simulink model "solver"  (R2022b)
settings: Solver=ode45  StartTime=0.0  StopTime=15.0  MaxStep=0.05  RelTol=1e-3
values from neighbouring files (symbols this model uses):
  Jb11 = m*(b^2+c^2)/12    (= 8.33333333333e-09)    [startup.m]
  Jb22 = m*(a^2+c^2)/12    (= 7.08333333333e-09)    [startup.m]
  Jb33 = m*(a^2+b^2)/12    (= 2.08333333333e-09)    [startup.m]
  Wx = Wxtilde*sqrt(0.99)    [startup.m]
  Wxtilde = sqrt((2*K)/Jb11)    [startup.m]
  Wy = Wytilde*sqrt(0.99)    [startup.m]
  Wz = Wztilde*sqrt(0.99)    [startup.m]
  Wztilde = 2*pi    (= 6.28318530718)    [startup.m]
libraries: vrlib x3
settings Model: Creator=eleves  LastModifiedBy=eleves

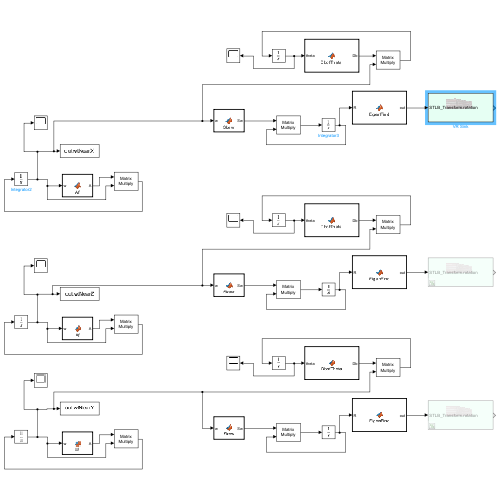
[thumbnail: Simulink's stored preview of the top-level diagram]
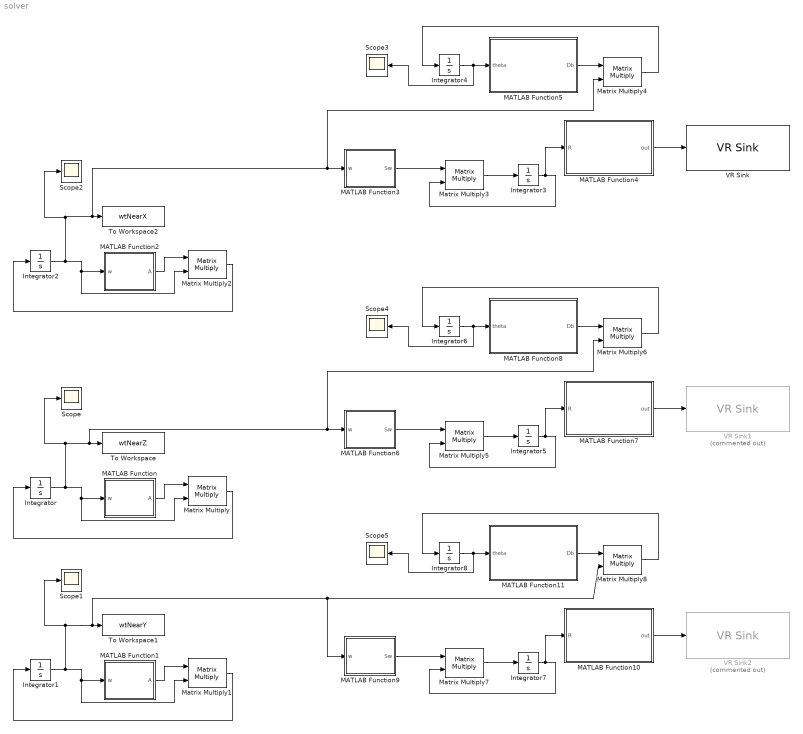
== system solver ==
  Integrator : Integrator  InitialCondition=[Wxtilde/10;0;Wz]
  Integrator1 : Integrator  InitialCondition=[0;Wy;Wztilde/10]
  Integrator2 : Integrator  InitialCondition=[Wx;0;Wztilde/10]
  Integrator3 : Integrator  InitialCondition=[1,0,0; 0,1,0; 0,0,1]
  Integrator4 : Integrator  InitialCondition=[0;0;0]
  Integrator5 : Integrator  InitialCondition=[1,0,0; 0,1,0; 0,0,1]
  Integrator6 : Integrator  InitialCondition=[0;0;0]
  Integrator7 : Integrator  InitialCondition=[1,0,0; 0,1,0; 0,0,1]
  Integrator8 : Integrator  InitialCondition=[0;0;0]
  MATLAB Function : MATLAB Function  TreatAsAtomicUnit=on
  MATLAB Function1 : MATLAB Function  TreatAsAtomicUnit=on
  MATLAB Function10 : MATLAB Function  TreatAsAtomicUnit=on
  MATLAB Function11 : MATLAB Function  TreatAsAtomicUnit=on
  MATLAB Function2 : MATLAB Function  TreatAsAtomicUnit=on
  MATLAB Function3 : MATLAB Function  TreatAsAtomicUnit=on
  MATLAB Function4 : MATLAB Function  TreatAsAtomicUnit=on
  MATLAB Function5 : MATLAB Function  TreatAsAtomicUnit=on
  MATLAB Function6 : MATLAB Function  TreatAsAtomicUnit=on
  MATLAB Function7 : MATLAB Function  TreatAsAtomicUnit=on
  MATLAB Function8 : MATLAB Function  TreatAsAtomicUnit=on
  MATLAB Function9 : MATLAB Function  TreatAsAtomicUnit=on
  Matrix Multiply{,1..8} (9 alike) : Product  Multiplication=Matrix(*)
  Scope{,1..5} (6 alike) : Scope
  To Workspace : ToWorkspace  VariableName=wtNearZ  SaveFormat=Timeseries  SampleTime=-1
  To Workspace1 : ToWorkspace  VariableName=wtNearY  SaveFormat=Timeseries  SampleTime=-1
  To Workspace2 : ToWorkspace  VariableName=wtNearX  SaveFormat=Timeseries  SampleTime=-1
  VR Sink : vrlib/VR Sink  InstantiateOnLoad=on  SampleTime=0.01  ViewEnable=on  RemoteChange=off  RemoteView=off  FieldsWritten=STLB_Transform.rotation.4.1.1.double  WorldFileName=test.x3d  AutoView=off  VideoDimensions=[200 320]  AllowVariableSize=off
  VR Sink1 : vrlib/VR Sink  Commented=on  InstantiateOnLoad=on  SampleTime=0.01  ViewEnable=on  RemoteChange=off  RemoteView=off  FieldsWritten=STLB_Transform.rotation.4.1.1.double  WorldFileName=test.x3d  AutoView=off  VideoDimensions=[200 320]  AllowVariableSize=off
  VR Sink2 : vrlib/VR Sink  Commented=on  InstantiateOnLoad=on  SampleTime=0.01  ViewEnable=on  RemoteChange=off  RemoteView=off  FieldsWritten=STLB_Transform.rotation.4.1.1.double  WorldFileName=test.x3d  AutoView=off  VideoDimensions=[200 320]  AllowVariableSize=off
  wires:
  MATLAB Function/1(A) -> Matrix Multiply/1
  Matrix Multiply/1 -> Integrator/1
  MATLAB Function1/1(A) -> Matrix Multiply1/1
  Matrix Multiply1/1 -> Integrator1/1
  Integrator2/1 -> Matrix Multiply4/2, MATLAB Function3/1(w), To Workspace2/1, Scope2/1, Matrix Multiply2/2, MATLAB Function2/1(w)
  MATLAB Function2/1(A) -> Matrix Multiply2/1
  Matrix Multiply2/1 -> Integrator2/1
  MATLAB Function3/1(Sw) -> Matrix Multiply3/1
  Matrix Multiply3/1 -> Integrator3/1
  Integrator3/1 -> MATLAB Function4/1(R), Matrix Multiply3/2
  MATLAB Function4/1(out) -> VR Sink/1
  Integrator4/1 -> Scope3/1, MATLAB Function5/1(theta)
  MATLAB Function5/1(Db) -> Matrix Multiply4/1
  Matrix Multiply4/1 -> Integrator4/1
  Integrator6/1 -> Scope4/1, MATLAB Function8/1(theta)
  MATLAB Function8/1(Db) -> Matrix Multiply6/1
  Matrix Multiply6/1 -> Integrator6/1
  MATLAB Function7/1(out) -> VR Sink1/1
  Integrator5/1 -> MATLAB Function7/1(R), Matrix Multiply5/2
  Integrator/1 -> Matrix Multiply6/2, MATLAB Function6/1(w), To Workspace/1, Scope/1, Matrix Multiply/2, MATLAB Function/1(w)
  Matrix Multiply5/1 -> Integrator5/1
  MATLAB Function6/1(Sw) -> Matrix Multiply5/1
  Integrator8/1 -> Scope5/1, MATLAB Function11/1(theta)
  MATLAB Function11/1(Db) -> Matrix Multiply8/1
  Matrix Multiply8/1 -> Integrator8/1
  MATLAB Function10/1(out) -> VR Sink2/1
  Integrator7/1 -> MATLAB Function10/1(R), Matrix Multiply7/2
  Integrator1/1 -> MATLAB Function9/1(w), Matrix Multiply8/2, To Workspace1/1, Scope1/1, Matrix Multiply1/2, MATLAB Function1/1(w)
  Matrix Multiply7/1 -> Integrator7/1
  MATLAB Function9/1(Sw) -> Matrix Multiply7/1

== matlab function solver/MATLAB Function1 ==
  data: w input; A output; Jb11 parameter; Jb22 parameter; Jb33 parameter
function A = Af(w, Jb11,Jb22, Jb33)

A = [0, (1/Jb11)*0.5*(Jb22-Jb33)*w(3),(1/Jb11)*0.5*(Jb22-Jb33)*w(2);
    (1/Jb22)*0.5*(Jb33-Jb11)*w(3),0,(1/Jb22)*0.5*(Jb33-Jb11)*w(1);
    (1/Jb33)*0.5*(Jb11-Jb22)*w(2),(1/Jb33)*0.5*(Jb11-Jb22)*w(1),0];

== matlab function solver/MATLAB Function ==
  data: w input; A output; Jb11 parameter; Jb22 parameter; Jb33 parameter
function A = Af(w, Jb11,Jb22, Jb33)

A = [0, (1/Jb11)*0.5*(Jb22-Jb33)*w(3),(1/Jb11)*0.5*(Jb22-Jb33)*w(2);
    (1/Jb22)*0.5*(Jb33-Jb11)*w(3),0,(1/Jb22)*0.5*(Jb33-Jb11)*w(1);
    (1/Jb33)*0.5*(Jb11-Jb22)*w(2),(1/Jb33)*0.5*(Jb11-Jb22)*w(1),0];

== matlab function solver/MATLAB Function2 ==
  data: w input; A output; Jb11 parameter; Jb22 parameter; Jb33 parameter
function A = Af(w, Jb11,Jb22, Jb33)

A = [0, (1/Jb11)*0.5*(Jb22-Jb33)*w(3),(1/Jb11)*0.5*(Jb22-Jb33)*w(2);
    (1/Jb22)*0.5*(Jb33-Jb11)*w(3),0,(1/Jb22)*0.5*(Jb33-Jb11)*w(1);
    (1/Jb33)*0.5*(Jb11-Jb22)*w(2),(1/Jb33)*0.5*(Jb11-Jb22)*w(1),0];

== matlab function solver/MATLAB Function3 ==
  data: w input; Sw output
function Sw = Skew(w)

Sw = [0,-w(3),w(2);
    w(3),0,-w(1);
    -w(2),w(1),0];

== matlab function solver/MATLAB Function4 ==
  data: R input; out output
function out = EigenFind(R)

    epsilon = 0.01; 
    epsilon2 = 0.1;
    
    if (abs(R(0+1,1+1)-R(1+1,0+1))< epsilon) && (abs(R(0+1,2+1)-R(2+1,0+1))< epsilon) && (abs(R(1+1,2+1)-R(2+1,1+1))< epsilon) 
	    % singularity found
	    % first check for identity matrix which must have +1 for all terms
	    %  in leading diagonaland zero in other terms
	    if (abs(R(0+1,1+1)+R(1+1,0+1)) < epsilon2) && (abs(R(0+1,2+1)+R(2+1,0+1)) < epsilon2) && (abs(R(1+1,2+1)+R(2+1,1+1)) < epsilon2) && (abs(R(0+1,0+1)+R(1+1,1+1)+R(2+1,2+1)-3) < epsilon2)
		    % this singularity is identity matrix so angle = 0
		    out= [1,0,0,0]; % zero angle, arbitrary axis
	    end
	    % otherwise this singularity is angle = 180
	    angle = pi;
	    xx = (R(0+1,0+1)+1)/2;
	    yy = (R(1+1,1+1)+1)/2;
	    zz = (R(2+1,2+1)+1)/2;
	    xy = (R(0+1,1+1)+R(1+1,0+1))/4;
	    xz = (R(0+1,2+1)+R(2+1,0+1))/4;
	    yz = (R(1+1,2+1)+R(2+1,1+1))/4;
	    if (xx > yy) && (xx > zz)  % R(0+1,0+1) is the largest diagonal term
		    if (xx< epsilon) 
			    x = 0;
			    y = 0.7071;
			    z = 0.7071;
		    else 
			    x = sqrt(xx);
			    y = xy/x;
			    z = xz/x;
		    end
    
	    elseif (yy > zz)  % R(1+1,1+1) is the largest diagonal term
		    if (yy< epsilon) 
			    x = 0.7071;
			    y = 0;
			    z = 0.7071;
		    else 
			    y = sqrt(yy);
			    x = xy/y;
			    z = yz/y;
		    end	
	    else  % R(2+1,2+1) is the largest diagonal term so base result on this
		    if (zz< epsilon) 
			    x = 0.7071;
			    y = 0.7071;
			    z = 0;
		    else 
			    z = sqrt(zz);
			    x = xz/z;
			    y = yz/z;
		    end
	    end
	    out = [x,y,z,angle]; % return 180 deg rotation
    end
    s = sqrt((R(2+1,1+1) - R(1+1,2+1))*(R(2+1,1+1) - R(1+1,2+1)) + (R(0+1,2+1) - R(2+1,0+1))*(R(0+1,2+1) - R(2+1,0+1)) + (R(1+1,0+1) - R(0+1,1+1))*(R(1+1,0+1) - R(0+1,1+1))); % used to normalise
    if (abs(s) < 0.001) 
	    s=1;
    end
    
	    % prevent divide by zero, should not happen if matrix is orthogonal and should be
	    % caught by singularity test above, but I ve left it in just in case
    angle = acos(( R(0+1,0+1) + R(1+1,1+1) + R(2+1,2+1) - 1)/2);
    x = (R(2+1,1+1) - R(1+1,2+1))/s;
    y = (R(0+1,2+1) - R(2+1,0+1))/s;
    z = (R(1+1,0+1) - R(0+1,1+1))/s;
    out = [x,y,z,angle];
end

== matlab function solver/MATLAB Function5 ==
  data: theta input; Db output
function Db = DbofTheta(theta)
    s1 = sin(theta(1));
    c1 = cos(theta(1));
    c2 = cos(theta(2)) ;
    t2 = tan(theta(2));
    Db = [1, s1*t2, c1*t2;
        0, c1, -s1;
        0 s1/c2, c1/c2];
end

== matlab function solver/MATLAB Function6 ==
  data: w input; Sw output
function Sw = Skew(w)

Sw = [0,-w(3),w(2);
    w(3),0,-w(1);
    -w(2),w(1),0];

== matlab function solver/MATLAB Function7 ==
  data: R input; out output
function out = EigenFind(R)

    epsilon = 0.01; 
    epsilon2 = 0.1;
    
    if (abs(R(0+1,1+1)-R(1+1,0+1))< epsilon) && (abs(R(0+1,2+1)-R(2+1,0+1))< epsilon) && (abs(R(1+1,2+1)-R(2+1,1+1))< epsilon) 
	    % singularity found
	    % first check for identity matrix which must have +1 for all terms
	    %  in leading diagonaland zero in other terms
	    if (abs(R(0+1,1+1)+R(1+1,0+1)) < epsilon2) && (abs(R(0+1,2+1)+R(2+1,0+1)) < epsilon2) && (abs(R(1+1,2+1)+R(2+1,1+1)) < epsilon2) && (abs(R(0+1,0+1)+R(1+1,1+1)+R(2+1,2+1)-3) < epsilon2)
		    % this singularity is identity matrix so angle = 0
		    out= [1,0,0,0]; % zero angle, arbitrary axis
	    end
	    % otherwise this singularity is angle = 180
	    angle = pi;
	    xx = (R(0+1,0+1)+1)/2;
	    yy = (R(1+1,1+1)+1)/2;
	    zz = (R(2+1,2+1)+1)/2;
	    xy = (R(0+1,1+1)+R(1+1,0+1))/4;
	    xz = (R(0+1,2+1)+R(2+1,0+1))/4;
	    yz = (R(1+1,2+1)+R(2+1,1+1))/4;
	    if (xx > yy) && (xx > zz)  % R(0+1,0+1) is the largest diagonal term
		    if (xx< epsilon) 
			    x = 0;
			    y = 0.7071;
			    z = 0.7071;
		    else 
			    x = sqrt(xx);
			    y = xy/x;
			    z = xz/x;
		    end
    
	    elseif (yy > zz)  % R(1+1,1+1) is the largest diagonal term
		    if (yy< epsilon) 
			    x = 0.7071;
			    y = 0;
			    z = 0.7071;
		    else 
			    y = sqrt(yy);
			    x = xy/y;
			    z = yz/y;
		    end	
	    else  % R(2+1,2+1) is the largest diagonal term so base result on this
		    if (zz< epsilon) 
			    x = 0.7071;
			    y = 0.7071;
			    z = 0;
		    else 
			    z = sqrt(zz);
			    x = xz/z;
			    y = yz/z;
		    end
	    end
	    out = [x,y,z,angle]; % return 180 deg rotation
    end
    s = sqrt((R(2+1,1+1) - R(1+1,2+1))*(R(2+1,1+1) - R(1+1,2+1)) + (R(0+1,2+1) - R(2+1,0+1))*(R(0+1,2+1) - R(2+1,0+1)) + (R(1+1,0+1) - R(0+1,1+1))*(R(1+1,0+1) - R(0+1,1+1))); % used to normalise
    if (abs(s) < 0.001) 
	    s=1;
    end
    
	    % prevent divide by zero, should not happen if matrix is orthogonal and should be
	    % caught by singularity test above, but I ve left it in just in case
    angle = acos(( R(0+1,0+1) + R(1+1,1+1) + R(2+1,2+1) - 1)/2);
    x = (R(2+1,1+1) - R(1+1,2+1))/s;
    y = (R(0+1,2+1) - R(2+1,0+1))/s;
    z = (R(1+1,0+1) - R(0+1,1+1))/s;
    out = [x,y,z,angle];
end

== matlab function solver/MATLAB Function8 ==
  data: theta input; Db output
function Db = DbofTheta(theta)
    s1 = sin(theta(1));
    c1 = cos(theta(1));
    c2 = cos(theta(2)) ;
    t2 = tan(theta(2));
    Db = [1, s1*t2, c1*t2;
        0, c1, -s1;
        0 s1/c2, c1/c2];
end

== matlab function solver/MATLAB Function10 ==
  data: R input; out output
function out = EigenFind(R)

    epsilon = 0.01; 
    epsilon2 = 0.1;
    
    if (abs(R(0+1,1+1)-R(1+1,0+1))< epsilon) && (abs(R(0+1,2+1)-R(2+1,0+1))< epsilon) && (abs(R(1+1,2+1)-R(2+1,1+1))< epsilon) 
	    % singularity found
	    % first check for identity matrix which must have +1 for all terms
	    %  in leading diagonaland zero in other terms
	    if (abs(R(0+1,1+1)+R(1+1,0+1)) < epsilon2) && (abs(R(0+1,2+1)+R(2+1,0+1)) < epsilon2) && (abs(R(1+1,2+1)+R(2+1,1+1)) < epsilon2) && (abs(R(0+1,0+1)+R(1+1,1+1)+R(2+1,2+1)-3) < epsilon2)
		    % this singularity is identity matrix so angle = 0
		    out= [1,0,0,0]; % zero angle, arbitrary axis
	    end
	    % otherwise this singularity is angle = 180
	    angle = pi;
	    xx = (R(0+1,0+1)+1)/2;
	    yy = (R(1+1,1+1)+1)/2;
	    zz = (R(2+1,2+1)+1)/2;
	    xy = (R(0+1,1+1)+R(1+1,0+1))/4;
	    xz = (R(0+1,2+1)+R(2+1,0+1))/4;
	    yz = (R(1+1,2+1)+R(2+1,1+1))/4;
	    if (xx > yy) && (xx > zz)  % R(0+1,0+1) is the largest diagonal term
		    if (xx< epsilon) 
			    x = 0;
			    y = 0.7071;
			    z = 0.7071;
		    else 
			    x = sqrt(xx);
			    y = xy/x;
			    z = xz/x;
		    end
    
	    elseif (yy > zz)  % R(1+1,1+1) is the largest diagonal term
		    if (yy< epsilon) 
			    x = 0.7071;
			    y = 0;
			    z = 0.7071;
		    else 
			    y = sqrt(yy);
			    x = xy/y;
			    z = yz/y;
		    end	
	    else  % R(2+1,2+1) is the largest diagonal term so base result on this
		    if (zz< epsilon) 
			    x = 0.7071;
			    y = 0.7071;
			    z = 0;
		    else 
			    z = sqrt(zz);
			    x = xz/z;
			    y = yz/z;
		    end
	    end
	    out = [x,y,z,angle]; % return 180 deg rotation
    end
    s = sqrt((R(2+1,1+1) - R(1+1,2+1))*(R(2+1,1+1) - R(1+1,2+1)) + (R(0+1,2+1) - R(2+1,0+1))*(R(0+1,2+1) - R(2+1,0+1)) + (R(1+1,0+1) - R(0+1,1+1))*(R(1+1,0+1) - R(0+1,1+1))); % used to normalise
    if (abs(s) < 0.001) 
	    s=1;
    end
    
	    % prevent divide by zero, should not happen if matrix is orthogonal and should be
	    % caught by singularity test above, but I ve left it in just in case
    angle = acos(( R(0+1,0+1) + R(1+1,1+1) + R(2+1,2+1) - 1)/2);
    x = (R(2+1,1+1) - R(1+1,2+1))/s;
    y = (R(0+1,2+1) - R(2+1,0+1))/s;
    z = (R(1+1,0+1) - R(0+1,1+1))/s;
    out = [x,y,z,angle];
end

== matlab function solver/MATLAB Function11 ==
  data: theta input; Db output
function Db = DbofTheta(theta)
    s1 = sin(theta(1));
    c1 = cos(theta(1));
    c2 = cos(theta(2)) ;
    t2 = tan(theta(2));
    Db = [1, s1*t2, c1*t2;
        0, c1, -s1;
        0 s1/c2, c1/c2];
end

== matlab function solver/MATLAB Function9 ==
  data: w input; Sw output
function Sw = Skew(w)

Sw = [0,-w(3),w(2);
    w(3),0,-w(1);
    -w(2),w(1),0];
